simulink model "problem4"  (R2020b)
settings: Solver=VariableStepAuto  StartTime=0.0  StopTime=10.0  RelTol=1e-3
settings Model: Creator=admin  LastModifiedBy=admin

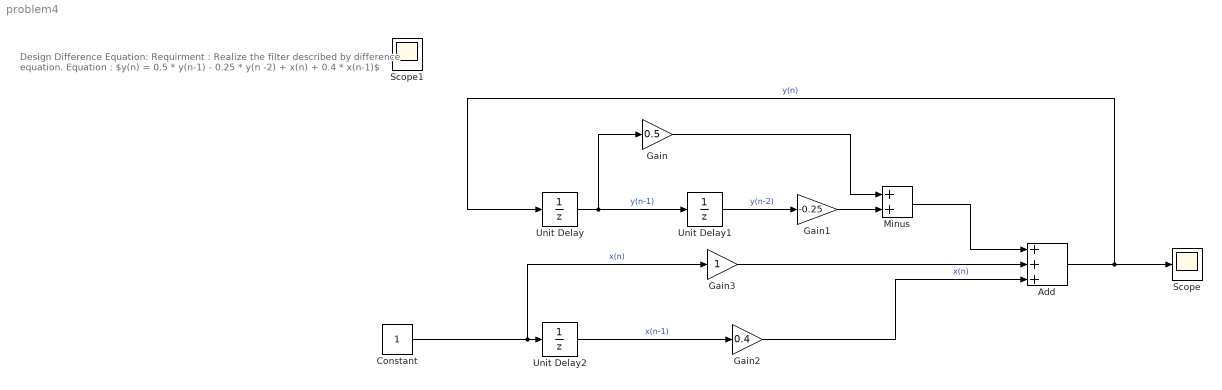
== system problem4 ==
  note: Design Difference Equation:
      |
      | Requirment :
      | Realize the filter described by difference equation.
      | Equation :
      | $y(n) = 0.5 * y(n-1) - 0.25 * y(n -2) + x(n) + 0.4 * x(n-1)$
  Add : Sum  Inputs=+++
  Constant : Constant
  Gain : Gain  Gain=0.5
  Gain1 : Gain  Gain=-0.25
  Gain2 : Gain  Gain=0.4
  Gain3 : Gain
  Minus : Sum
  Scope : Scope
  Unit Delay : UnitDelay  SampleTime=-1  HasFrameUpgradeWarning=on
  Unit Delay1 : UnitDelay  SampleTime=-1  HasFrameUpgradeWarning=on
  Unit Delay2 : UnitDelay  SampleTime=-1  HasFrameUpgradeWarning=on
  Scope1 : Scope
  wires:
  Unit Delay/1 -> Gain/1, Unit Delay1/1  "y(n-1)"
  Unit Delay1/1 -> Gain1/1  "y(n-2)"
  Unit Delay2/1 -> Gain2/1  "x(n-1)"
  Constant/1 -> Gain3/1, Unit Delay2/1  "x(n)"
  Gain2/1 -> Add/3  "x(n)"
  Gain1/1 -> Minus/2
  Gain/1 -> Minus/1
  Minus/1 -> Add/1
  Add/1 -> Unit Delay/1, Scope/1  "y(n)"
  Gain3/1 -> Add/2
